simulink model "Batterytempandcapacityeffect"  (R2021b)
settings: Solver=ode45  StartTime=0.0  StopTime=25000  RelTol=1e-3  EnableMultiTasking=on
undefined symbols (not defined in the file): sigbuilder_block
settings Model: Creator=Shivraj  LastModifiedBy=Shiv
settings SolverCC: AlgebraicLoopSolver=TrustRegion
settings DataIOCC: LimitDataPoints=on  SaveFormat=Array  ReturnWorkspaceOutputs=off
settings OptimizationCC: LifeSpan=inf
settings DebuggingCC: SFUnexpectedBacktrackingDiag=warning  SFNoUnconditionalDefaultTransitionDiag=warning  SFExecutionAtInitializationDiag=none  SFMachineParentedDataDiag=warning  ArithmeticOperatorsInVariantConditions=warning
settings HardwareCC: ProdBitPerPointer=32  ProdBitPerSizeT=32  ProdBitPerPtrDiffT=32  ProdLargestAtomicFloat=None  ProdIntDivRoundTo=Undefined  ProdEndianess=Unspecified  ProdWordSize=32  ProdHWDeviceType=32-bit Generic
settings ModelReferenceCC: PropagateSignalLabelsOutOfModel=off
settings SFSimCC: SimUseLocalCustomCode=off  CustomCodeUndefinedFunction=UseInterfaceOnly
settings RTWCC: RTWUseLocalCustomCode=off
settings CodeAppCC: StateflowObjectComments=on
settings GRTTargetCC: TargetLangStandard=C89/C90 (ANSI)
settings ConfigComp: CovMetricSettings=dw  CovSaveCumulativeToWorkspaceVar=on  CovSaveSingleToWorkspaceVar=on  CovExternalEMLEnable=off  CovSFcnEnable=off

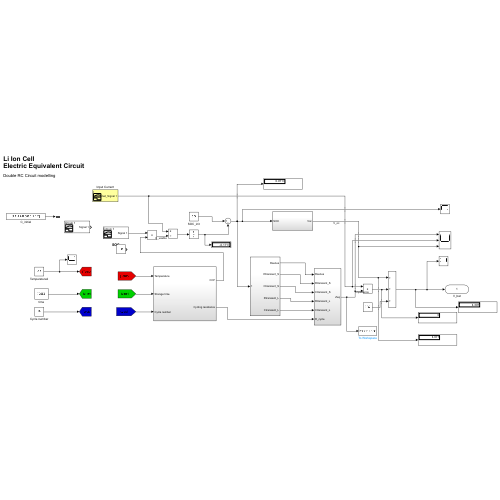
[thumbnail: Simulink's stored preview of the top-level diagram]
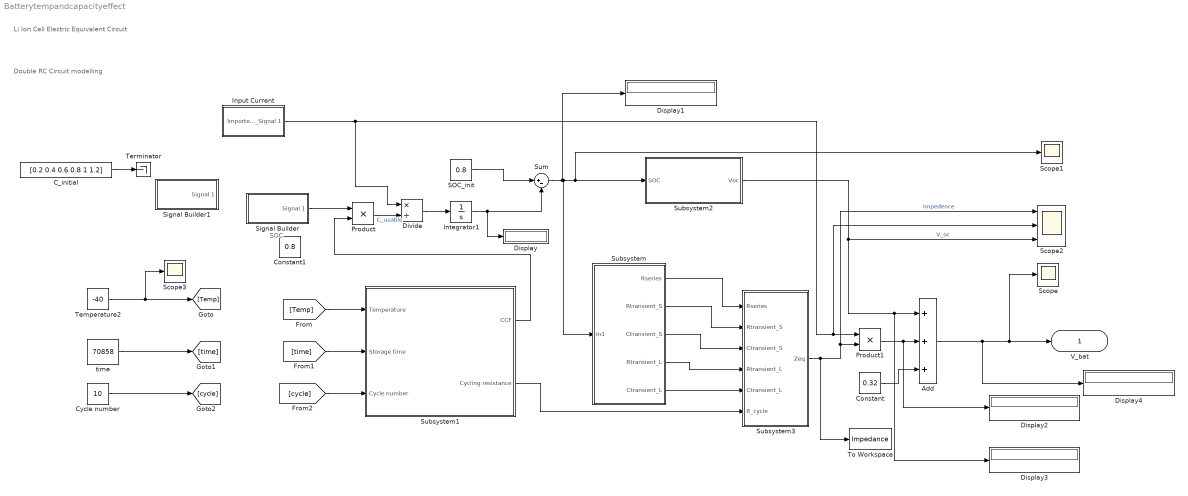
== system Batterytempandcapacityeffect ==
  note: SOC
  note: Double RC Circuit modelling
  note: Li Ion Cell
      | Electric Equivalent Circuit
  Add : Sum  Inputs=+++
  C_initial : Constant  Value=[0.2 0.4 0.6 0.8 1 1.2]
  Constant : Constant  Value=0.32
  Constant1 : Constant  Value=0.8
  Cycle number : Constant  Value=10
  Display{,1..4} (5 alike) : Display
  Divide : Product  Inputs=*/
  Input Current : Subsystem  Tag=STV Subsys  LoadFcn=sigbuilder_block('load');  StartFcn=sigbuilder_block('start');  StopFcn=sigbuilder_block('stop');  ClipboardFcn=sigbuilder_block('clipboard');  mask(Sigbuilder block){tuvar=[0:10]}
      mask help: Simulink:masks:SigbuilderBlock_MD
      mask init:
      | if ~strcmp(get_param(bdroot(gcbh),'SimulationStatus'),'stopped') tuvar = sigbuilder_block('maskInit'); end
      settings: CopyFcn=sigbuilder_block('copy');  DeleteFcn=sigbuilder_block('delete');  ModelCloseFcn=sigbuilder_block('modelClose');  PreSaveFcn=sigbuilder_block('preSave');  PauseFcn=sigbuilder_block('pause');  ContinueFcn=sigbuilder_block('continue');  NameChangeFcn=sigbuilder_block('namechange');  OpenFcn=sigbuilder_block('open',[6 51 1012.5 460.5 ]);  CloseFcn=sigbuilder_block('close');
      mask Display: plot(0, 0, 100, 100,[2, 2, 32, 32, 2], [68, 8, 8, 68, 68],[32, 2], [38, 38], [32, 19, 2],[53, 60, 44], [32, 17, 17, 2],[16, 16, 31, 31]);txt = getActiveGroup(gcbh);text(2, 100, txt,'verticalAlignment', 'top');
  Integrator1 : Integrator  UpperSaturationLimit=100  LowerSaturationLimit=0
  Product : Product
  Product1 : Product
  SOC_init : Constant  Value=0.8
  Scope : Scope
  Scope1 : Scope
  Scope2 : Scope  NumInputPorts=3
  Scope3 : Scope
  Signal Builder : Subsystem  Tag=STV Subsys  LoadFcn=sigbuilder_block('load');  StartFcn=sigbuilder_block('start');  StopFcn=sigbuilder_block('stop');  ClipboardFcn=sigbuilder_block('clipboard');  mask(Sigbuilder block){tuvar=[0:10]}
      mask help: Simulink:masks:SigbuilderBlock_MD
      mask init:
      | if ~strcmp(get_param(bdroot(gcbh),'SimulationStatus'),'stopped') tuvar = sigbuilder_block('maskInit'); end
      settings: CopyFcn=sigbuilder_block('copy');  DeleteFcn=sigbuilder_block('delete');  ModelCloseFcn=sigbuilder_block('modelClose');  PreSaveFcn=sigbuilder_block('preSave');  PauseFcn=sigbuilder_block('pause');  ContinueFcn=sigbuilder_block('continue');  NameChangeFcn=sigbuilder_block('namechange');  OpenFcn=sigbuilder_block('open',[205.5 54 550.5 359.25 ]);  CloseFcn=sigbuilder_block('close');
      mask Display: plot(0, 0, 100, 100,[2, 2, 32, 32, 2], [68, 8, 8, 68, 68],[32, 2], [38, 38], [32, 19, 2],[53, 60, 44], [32, 17, 17, 2],[16, 16, 31, 31]);txt = getActiveGroup(gcbh);text(2, 100, txt,'verticalAlignment', 'top');
  Signal Builder1 : Subsystem  Tag=STV Subsys  LoadFcn=sigbuilder_block('load');  StartFcn=sigbuilder_block('start');  StopFcn=sigbuilder_block('stop');  ClipboardFcn=sigbuilder_block('clipboard');  mask(Sigbuilder block){tuvar=[0:10]}
      mask help: Simulink:masks:SigbuilderBlock_MD
      mask init:
      | if ~strcmp(get_param(bdroot(gcbh),'SimulationStatus'),'stopped') tuvar = sigbuilder_block('maskInit'); end
      settings: CopyFcn=sigbuilder_block('copy');  DeleteFcn=sigbuilder_block('delete');  ModelCloseFcn=sigbuilder_block('modelClose');  PreSaveFcn=sigbuilder_block('preSave');  PauseFcn=sigbuilder_block('pause');  ContinueFcn=sigbuilder_block('continue');  NameChangeFcn=sigbuilder_block('namechange');  OpenFcn=sigbuilder_block('open',[437.6 153 550.4 359.25 ]);  CloseFcn=sigbuilder_block('close');
      mask Display: plot(0, 0, 100, 100,[2, 2, 32, 32, 2], [68, 8, 8, 68, 68],[32, 2], [38, 38], [32, 19, 2],[53, 60, 44], [32, 17, 17, 2],[16, 16, 31, 31]);txt = getActiveGroup(gcbh);text(2, 100, txt,'verticalAlignment', 'top');
  Subsystem : Subsystem
  Subsystem1 : Subsystem
  Subsystem2 : Subsystem
  Subsystem3 : Subsystem
  Sum : Sum  Inputs=|+-
  Temperature2 : Constant  Value=-40
  Terminator : Terminator
  To Workspace : ToWorkspace  VariableName=Impedance  SaveFormat=Timeseries  SampleTime=-1
      settings: MaxDataPoints=25000
  "time " : Constant  Value=70858
  "V_bat " : Outport  VectorParamsAs1DForOutWhenUnconnected=off
  wires:
  Subsystem1/1(CCF) -> Product/2
  Product/1 -> Divide/2  "C_usable"
  Input Current/1(Imported_Signal 1) -> Divide/1, Scope2/2, Product1/1
  SOC_init/1 -> Sum/1
  Sum/1 -> Subsystem2/1(SOC), Scope1/1, Subsystem/1(In1), Display1/1
  Subsystem3/1(Zeq) -> To Workspace/1, Scope2/1, Product1/2  "Impedence"
  Product1/1 -> Display2/1, Add/2
  Subsystem2/1(Voc) -> Scope2/3, Display3/1, Add/1  "V_oc"
  Subsystem/1(Rseries) -> Subsystem3/1(Rseries)
  Subsystem/2(Rtransient_S) -> Subsystem3/2(Rtransient_S)
  Subsystem/3(Ctransient_S) -> Subsystem3/3(Ctransient_S)
  Subsystem/4(Rtransient_L) -> Subsystem3/4(Rtransient_L)
  Subsystem/5(Ctransient_L) -> Subsystem3/5(Ctransient_L)
  Subsystem1/2(Cycling resistance) -> Subsystem3/6(R_cycle)
  Add/1 -> Display4/1, Scope/1, "V_bat "/1
  Temperature2/1 -> Scope3/1, [Temp]
  "time "/1 -> [time]
  Cycle number/1 -> [cycle]
  [Temp] -> Subsystem1/1(Temperature)
  [time] -> Subsystem1/2(Storage time)
  [cycle] -> Subsystem1/3(Cycle number)
  Divide/1 -> Integrator1/1
  Integrator1/1 -> Sum/2, Display/1
  C_initial/1 -> Terminator/1
  Constant/1 -> Add/3
  Signal Builder/1(Signal 1) -> Product/1

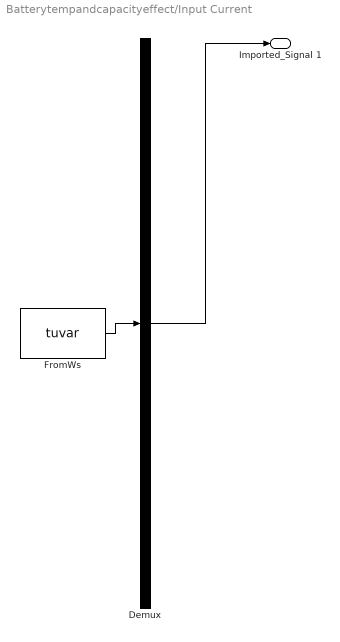
== system Batterytempandcapacityeffect/Input Current ==
  Demux : Demux  Tag=STV Demux  Outputs=1
      settings: DisplayOption=none
  FromWs : FromWorkspace  Tag=STV FromWs  VariableName=tuvar
      SigBuilderData=|
      | common.afterFinalStr = 'Extrapolate'
      | common.sampleTime = 0
      | dataSet.timeRange = [0 22502.2]
      | dataSet.name = 'I'
      | sbobj.Name = 'Signal Builder'
      | sbobj.Groups.Name = 'I'
      | sbobj.Groups.Signals.Name = 'Imported_Signal 1'
      | sbobj.Groups.Signals.XData = [0 0.05 0.1 0.15 0.2 0.25 0.3 0.35 0.4 0.45 0.5 0.55 ... (450045 elements, 1x450045)]
      | sbobj.Groups.Signals.YData = [0 0 0 0 0 0 0 0 0 0 0 0 ... (450045 elements, 1x450045)]
      | sbobj.Groups.TimeRange = [0 22502.2]
  Imported_Signal 1 : Outport  VectorParamsAs1DForOutWhenUnconnected=off
  wires:
  Demux/1 -> Imported_Signal 1/1
  FromWs/1 -> Demux/1

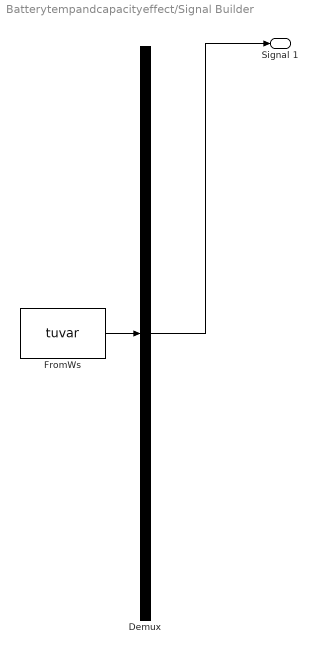
== system Batterytempandcapacityeffect/Signal Builder ==
  Demux : Demux  Tag=STV Demux  Outputs=1
      settings: DisplayOption=none
  FromWs : FromWorkspace  Tag=STV FromWs  VariableName=tuvar
      SigBuilderData=|
      | common.afterFinalStr = 'Extrapolate'
      | common.sampleTime = 0
      | dataSet.timeRange = [0 10]
      | dataSet.name = 'Group 1'
      | sbobj.Groups.Name = 'Group 1'
      | sbobj.Groups.Signals.Name = 'Signal 1'
      | sbobj.Groups.Signals.XData = [0 2 2.5 4 4.5 6 8 10]
      | sbobj.Groups.Signals.YData = [1.09 0.925 0.805 0.73 0.585 0.465 0.26 0.175]
  Signal 1 : Outport  Tag=STV Outport  VectorParamsAs1DForOutWhenUnconnected=off
  wires:
  Demux/1 -> Signal 1/1
  FromWs/1 -> Demux/1

== system Batterytempandcapacityeffect/Signal Builder1 ==
  Demux : Demux  Tag=STV Demux  Outputs=1
      settings: DisplayOption=none
  FromWs : FromWorkspace  Tag=STV FromWs  VariableName=tuvar
      SigBuilderData=|
      | common.afterFinalStr = 'Extrapolate'
      | common.sampleTime = 0
      | dataSet.timeRange = [0 10]
      | dataSet.name = 'Group 1'
      | sbobj.Groups.Name = 'Group 1'
      | sbobj.Groups.Signals.Name = 'Signal 1'
      | sbobj.Groups.Signals.XData = [0 1 2 2.5 3 3.5 4 4.5 6 8 10]
      | sbobj.Groups.Signals.YData = [0.175 0.295 0.41 0.53 0.675 0.74 0.82 0.88 1.03 1.12 1.175]
  Signal 1 : Outport  Tag=STV Outport  VectorParamsAs1DForOutWhenUnconnected=off
  wires:
  FromWs/1 -> Demux/1
  Demux/1 -> Signal 1/1

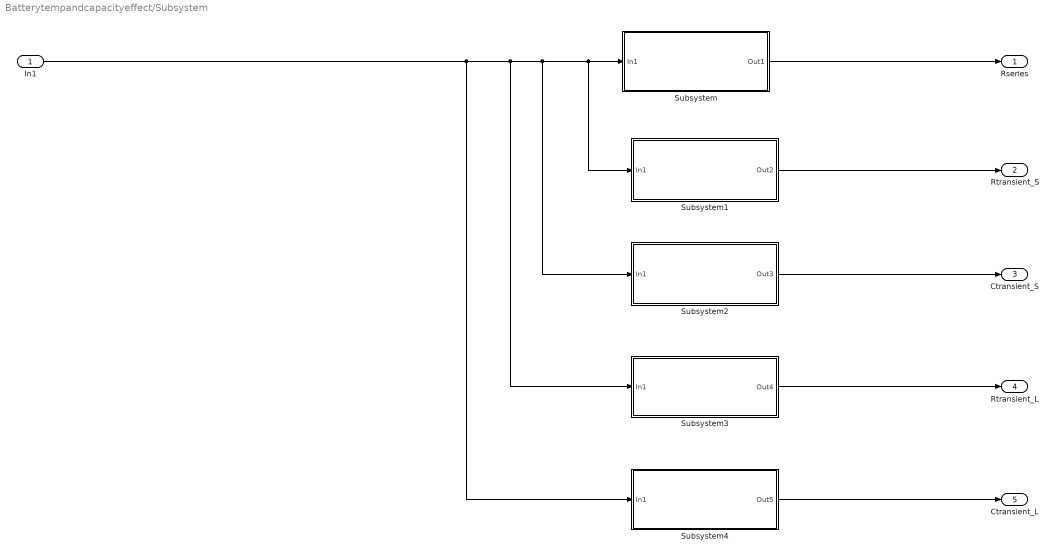
== system Batterytempandcapacityeffect/Subsystem ==
  In1 : Inport
  Subsystem : Subsystem
  Subsystem1 : Subsystem
  Subsystem2 : Subsystem
  Subsystem3 : Subsystem
  Subsystem4 : Subsystem
  Rseries : Outport  VectorParamsAs1DForOutWhenUnconnected=off
  Rtransient_S : Outport  Port=2  VectorParamsAs1DForOutWhenUnconnected=off
  Ctransient_S : Outport  Port=3  VectorParamsAs1DForOutWhenUnconnected=off
  Rtransient_L : Outport  Port=4  VectorParamsAs1DForOutWhenUnconnected=off
  Ctransient_L : Outport  Port=5  VectorParamsAs1DForOutWhenUnconnected=off
  wires:
  In1/1 -> Subsystem4/1(In1), Subsystem3/1(In1), Subsystem2/1(In1), Subsystem1/1(In1), Subsystem/1(In1)
  Subsystem/1(Out1) -> Rseries/1
  Subsystem1/1("Out2 ") -> Rtransient_S/1
  Subsystem2/1(Out3) -> Ctransient_S/1
  Subsystem3/1("Out4 ") -> Rtransient_L/1
  Subsystem4/1("Out5 ") -> Ctransient_L/1

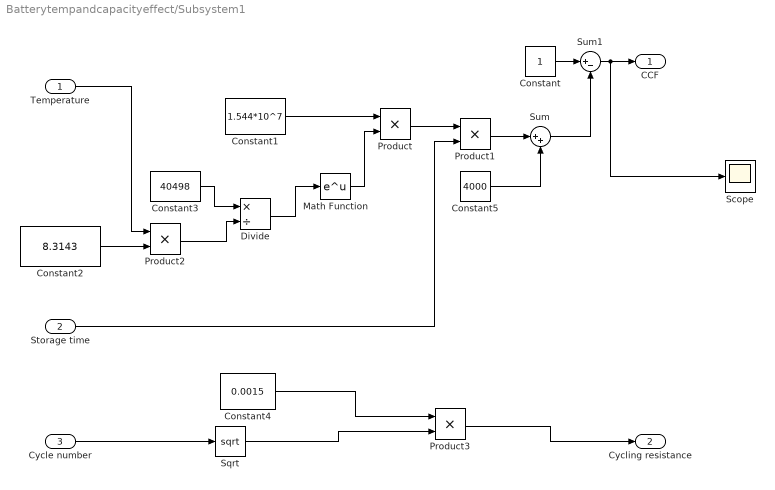
== system Batterytempandcapacityeffect/Subsystem1 ==
  Temperature : Inport
  Storage time : Inport  Port=2
  Cycle number : Inport  Port=3
  Constant : Constant
  Constant1 : Constant  Value=1.544*10^7
  Constant2 : Constant  Value=8.3143
  Constant3 : Constant  Value=40498
  Constant4 : Constant  Value=0.0015
  Constant5 : Constant  Value=4000
  Divide : Product  Inputs=*/
  Math Function : Math  SignedPower=on  SaturateOnIntegerOverflow=on
  Product{,1..3} (4 alike) : Product
  Scope : Scope
  Sqrt : Sqrt  SaturateOnIntegerOverflow=on
  Sum : Sum  Inputs=|++
  Sum1 : Sum  Inputs=|+-
  CCF : Outport  VectorParamsAs1DForOutWhenUnconnected=off
  Cycling resistance : Outport  Port=2  VectorParamsAs1DForOutWhenUnconnected=off
  wires:
  Sum/1 -> Sum1/2
  Constant/1 -> Sum1/1
  Sum1/1 -> Scope/1, CCF/1
  Constant1/1 -> Product/1
  Math Function/1 -> Product/2
  Product/1 -> Product1/1
  Storage time/1 -> Product1/2
  Constant2/1 -> Product2/2
  Temperature/1 -> Product2/1
  Divide/1 -> Math Function/1
  Constant3/1 -> Divide/1
  Product2/1 -> Divide/2
  Cycle number/1 -> Sqrt/1
  Constant4/1 -> Product3/1
  Sqrt/1 -> Product3/2
  Product3/1 -> Cycling resistance/1
  Product1/1 -> Sum/1
  Constant5/1 -> Sum/2

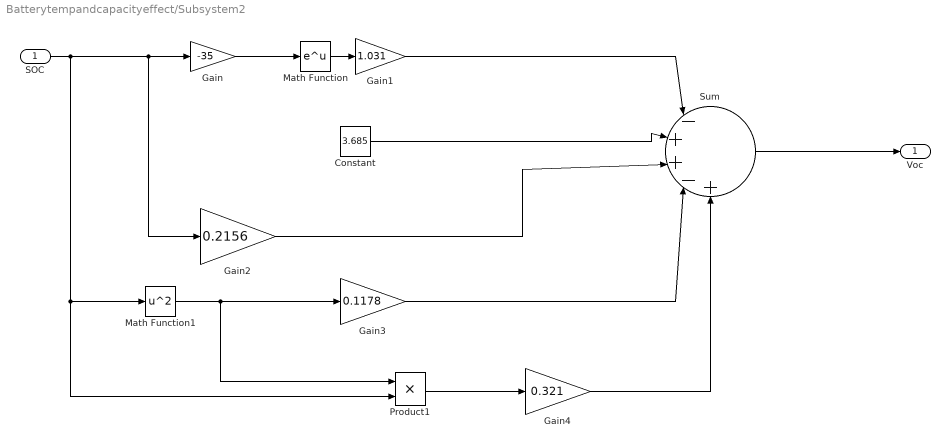
== system Batterytempandcapacityeffect/Subsystem2 ==
  SOC : Inport
  Constant : Constant  Value=3.685
  Gain : Gain  Gain=-35
  Gain1 : Gain  Gain=1.031
  Gain2 : Gain  Gain=0.2156
  Gain3 : Gain  Gain=0.1178
  Gain4 : Gain  Gain=0.321
  Math Function : Math  SignedPower=on  SaturateOnIntegerOverflow=on
  Math Function1 : Math  Operator=square  SignedPower=on  SaturateOnIntegerOverflow=on
  Product1 : Product
  Sum : Sum  Inputs=|-++-+
  Voc : Outport  VectorParamsAs1DForOutWhenUnconnected=off
  wires:
  Math Function/1 -> Gain1/1
  Constant/1 -> Sum/2
  Gain1/1 -> Sum/1
  Gain/1 -> Math Function/1
  Gain2/1 -> Sum/3
  Math Function1/1 -> Product1/1, Gain3/1
  Gain3/1 -> Sum/4
  Product1/1 -> Gain4/1
  Gain4/1 -> Sum/5
  Sum/1 -> Voc/1
  SOC/1 -> Product1/2, Math Function1/1, Gain2/1, Gain/1

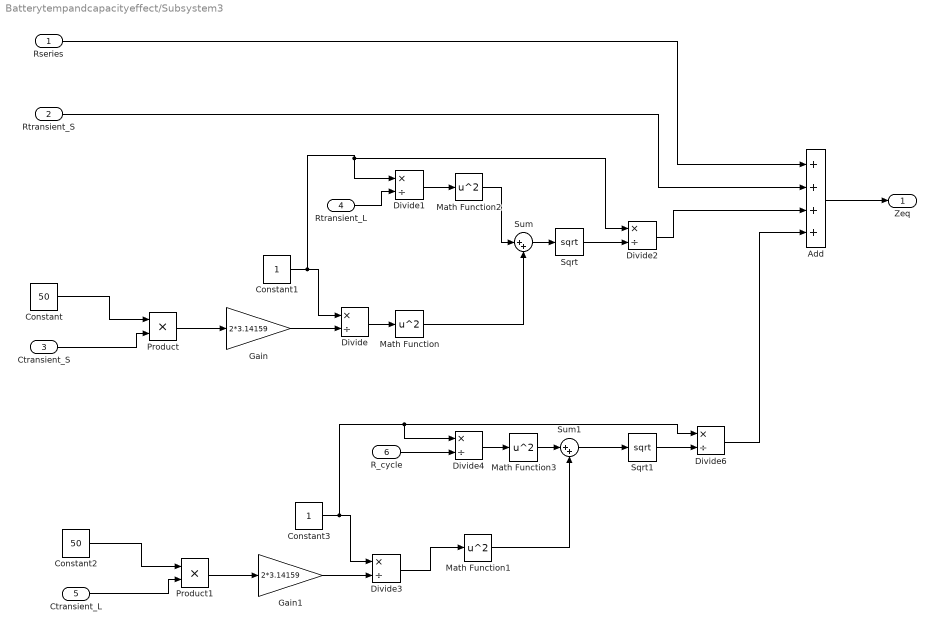
== system Batterytempandcapacityeffect/Subsystem3 ==
  Rseries : Inport
  Rtransient_S : Inport  Port=2
  Ctransient_S : Inport  Port=3
  Rtransient_L : Inport  Port=4
  Ctransient_L : Inport  Port=5
  R_cycle : Inport  Port=6
  Add : Sum  Inputs=++++
  Constant : Constant  Value=50
  Constant1 : Constant
  Constant2 : Constant  Value=50
  Constant3 : Constant
  Divide{,1..4,6} (6 alike) : Product  Inputs=*/
  Gain : Gain  Gain=2*3.14159
  Gain1 : Gain  Gain=2*3.14159
  Math Function{,1..3} (4 alike) : Math  Operator=square  SignedPower=on  SaturateOnIntegerOverflow=on
  Product : Product
  Product1 : Product
  Sqrt : Sqrt  SaturateOnIntegerOverflow=on
  Sqrt1 : Sqrt  SaturateOnIntegerOverflow=on
  Sum : Sum  Inputs=|++
  Sum1 : Sum  Inputs=|++
  Zeq : Outport  VectorParamsAs1DForOutWhenUnconnected=off
  wires:
  Add/1 -> Zeq/1
  Rseries/1 -> Add/1
  Rtransient_S/1 -> Add/2
  Ctransient_S/1 -> Product/2
  Constant/1 -> Product/1
  Product/1 -> Gain/1
  Gain/1 -> Divide/2
  Constant1/1 -> Divide2/1, Divide1/1, Divide/1
  Rtransient_L/1 -> Divide1/2
  Divide/1 -> Math Function/1
  Math Function/1 -> Sum/2
  Divide1/1 -> Math Function2/1
  Math Function2/1 -> Sum/1
  Sum/1 -> Sqrt/1
  Sqrt/1 -> Divide2/2
  Ctransient_L/1 -> Product1/2
  Constant2/1 -> Product1/1
  Product1/1 -> Gain1/1
  Gain1/1 -> Divide3/2
  Constant3/1 -> Divide3/1, Divide4/1, Divide6/1
  R_cycle/1 -> Divide4/2
  Divide3/1 -> Math Function1/1
  Math Function1/1 -> Sum1/2
  Divide4/1 -> Math Function3/1
  Math Function3/1 -> Sum1/1
  Sum1/1 -> Sqrt1/1
  Divide2/1 -> Add/3
  Sqrt1/1 -> Divide6/2
  Divide6/1 -> Add/4

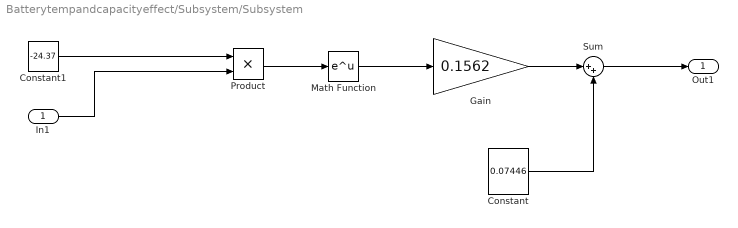
== system Batterytempandcapacityeffect/Subsystem/Subsystem ==
  In1 : Inport
  Constant : Constant  Value=0.07446
  Constant1 : Constant  Value=-24.37
  Gain : Gain  Gain=0.1562
  Math Function : Math  SignedPower=on  SaturateOnIntegerOverflow=on
  Product : Product
  Sum : Sum  Inputs=|++
  Out1 : Outport  VectorParamsAs1DForOutWhenUnconnected=off
  wires:
  Sum/1 -> Out1/1
  Product/1 -> Math Function/1
  Constant/1 -> Sum/2
  Math Function/1 -> Gain/1
  In1/1 -> Product/2
  Constant1/1 -> Product/1
  Gain/1 -> Sum/1

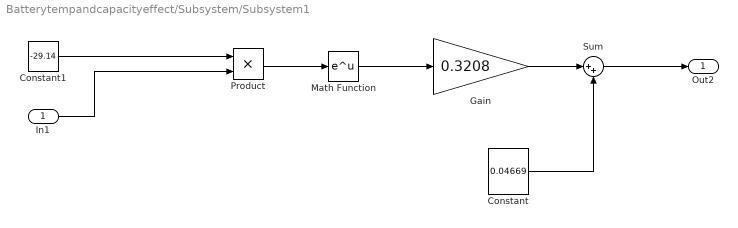
== system Batterytempandcapacityeffect/Subsystem/Subsystem1 ==
  In1 : Inport
  Constant : Constant  Value=0.04669
  Constant1 : Constant  Value=-29.14
  Gain : Gain  Gain=0.3208
  Math Function : Math  SignedPower=on  SaturateOnIntegerOverflow=on
  Product : Product
  Sum : Sum  Inputs=|++
  "Out2 " : Outport  VectorParamsAs1DForOutWhenUnconnected=off
  wires:
  Gain/1 -> Sum/1
  Constant1/1 -> Product/1
  In1/1 -> Product/2
  Math Function/1 -> Gain/1
  Constant/1 -> Sum/2
  Product/1 -> Math Function/1
  Sum/1 -> "Out2 "/1

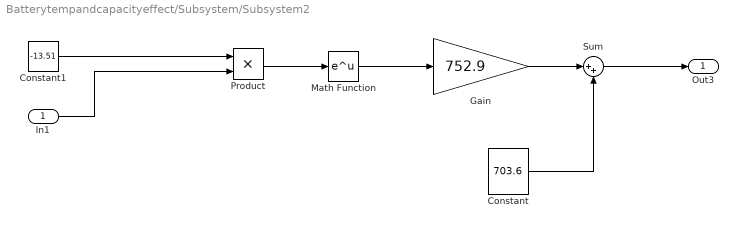
== system Batterytempandcapacityeffect/Subsystem/Subsystem2 ==
  In1 : Inport
  Constant : Constant  Value=703.6
  Constant1 : Constant  Value=-13.51
  Gain : Gain  Gain=752.9
  Math Function : Math  SignedPower=on  SaturateOnIntegerOverflow=on
  Product : Product
  Sum : Sum  Inputs=|++
  Out3 : Outport  VectorParamsAs1DForOutWhenUnconnected=off
  wires:
  Sum/1 -> Out3/1
  Product/1 -> Math Function/1
  Constant/1 -> Sum/2
  Math Function/1 -> Gain/1
  In1/1 -> Product/2
  Constant1/1 -> Product/1
  Gain/1 -> Sum/1

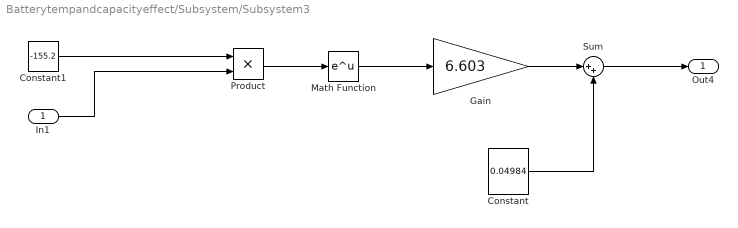
== system Batterytempandcapacityeffect/Subsystem/Subsystem3 ==
  In1 : Inport
  Constant : Constant  Value=0.04984
  Constant1 : Constant  Value=-155.2
  Gain : Gain  Gain=6.603
  Math Function : Math  SignedPower=on  SaturateOnIntegerOverflow=on
  Product : Product
  Sum : Sum  Inputs=|++
  "Out4 " : Outport  VectorParamsAs1DForOutWhenUnconnected=off
  wires:
  Gain/1 -> Sum/1
  Constant1/1 -> Product/1
  In1/1 -> Product/2
  Math Function/1 -> Gain/1
  Constant/1 -> Sum/2
  Product/1 -> Math Function/1
  Sum/1 -> "Out4 "/1

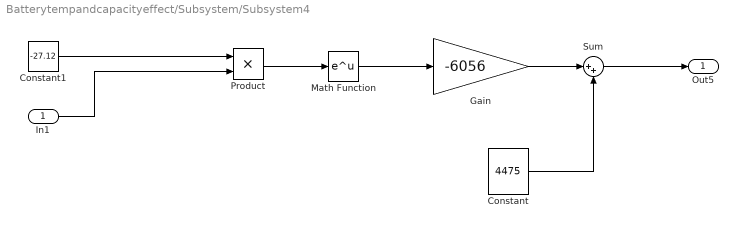
== system Batterytempandcapacityeffect/Subsystem/Subsystem4 ==
  In1 : Inport
  Constant : Constant  Value=4475
  Constant1 : Constant  Value=-27.12
  Gain : Gain  Gain=-6056
  Math Function : Math  SignedPower=on  SaturateOnIntegerOverflow=on
  Product : Product
  Sum : Sum  Inputs=|++
  "Out5 " : Outport  VectorParamsAs1DForOutWhenUnconnected=off
  wires:
  Sum/1 -> "Out5 "/1
  Product/1 -> Math Function/1
  Constant/1 -> Sum/2
  Math Function/1 -> Gain/1
  In1/1 -> Product/2
  Constant1/1 -> Product/1
  Gain/1 -> Sum/1
